simulink model "singleStepPredict"  (R2018a)
settings: Solver=VariableStepAuto  StartTime=0.0  StopTime=0.1  RelTol=1e-3
values from neighbouring files (symbols this model uses):
  c_theta = d_theta(n) * pi / 180    [old_PlotFigure.m]
  fai = yaw(n) * pi /180    [old_PlotFigure.m]
  l = 1.06    [old_PlotFigure.m]
  lb = calculFai(n)    [old_PlotFigure.m]
  ub = c_theta    [old_PlotFigure.m]
  v = vmid    (= 0.3402)    [old_PlotFigure.m]
  v_theta = -front_wheel_angle_spd    (= -3.3879920774)    [old_PlotFigure.m]
settings Model: Creator=18428  LastModifiedBy=Administrator

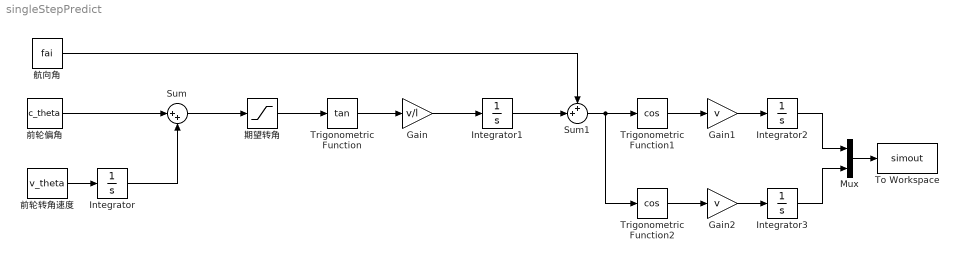
== system singleStepPredict ==
  Gain : Gain  Gain=v/l
  Gain1 : Gain  Gain=v
  Gain2 : Gain  Gain=v
  Integrator{,1..3} (4 alike) : Integrator
  Mux : Mux  Inputs=2
  Sum : Sum  Inputs=|++
  Sum1 : Sum  Inputs=++|
  To Workspace : ToWorkspace  VariableName=simout  SaveFormat=Timeseries  SampleTime=-1
  Trigonometric Function : Trigonometry  Operator=tan
  Trigonometric Function1 : Trigonometry  Operator=cos
  Trigonometric Function2 : Trigonometry  Operator=cos
  前轮偏角 : Constant  Value=c_theta
  前轮转角速度 : Constant  Value=v_theta
  期望转角 : Saturate  UpperLimit=ub  LowerLimit=lb
  航向角 : Constant  Value=fai
  wires:
  前轮偏角/1 -> Sum/1
  Sum/1 -> 期望转角/1
  前轮转角速度/1 -> Integrator/1
  Integrator/1 -> Sum/2
  期望转角/1 -> Trigonometric Function/1
  Trigonometric Function/1 -> Gain/1
  Gain/1 -> Integrator1/1
  Integrator1/1 -> Sum1/2
  航向角/1 -> Sum1/1
  Trigonometric Function1/1 -> Gain1/1
  Gain1/1 -> Integrator2/1
  Integrator3/1 -> Mux/2
  Gain2/1 -> Integrator3/1
  Trigonometric Function2/1 -> Gain2/1
  Sum1/1 -> Trigonometric Function2/1, Trigonometric Function1/1
  Integrator2/1 -> Mux/1
  Mux/1 -> To Workspace/1
